simulink library "lib_Convection_FCConcCyls"  (R2015a)
settings: Solver=ode45  StartTime=0.0  StopTime=10.0  RelTol=1e-3
libraries: simulink x5, lib_Convection_NonDimParms x1
settings Model: Creator=jlkratz  LastModifiedBy=jlkratz

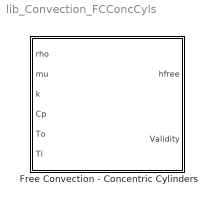
== system lib_Convection_FCConcCyls ==
  Free Convection - Concentric Cylinders : Subsystem  mask(TSAT: Concentric Cylinders Free Convection){R_M=1716, g_M=32.174, Ro_M=[1.5 5], Ri_M=[1 4], InOrOutSurf_M=Inner Surface}
      mask prompts: R_M "R_M - Real gas constant"; g_M "g_M - Acceleration due to gravity"; Ro_M "Ro_M - Radius of the outer cylinder"; Ri_M "Ri_M - Radius of the inner cylinder"; InOrOutSurf_M "InOrOutSurf_M - Select surface"
      mask help:
      | This block estimates the average convective heat transfer coefficient for free convection within concentric cylinders for either the inner or outer surface. The employed correlation is the work of Raithby and Hollands. Note that all fluid properrties should be evaluated at average of the hot and cold surface. To get the heat flux for the selected inner or outer surface, multiply the output (h) by the difference in temperature between the opposite surface and the selected surface. This number may be negative. Restrictions to the implemented correlation includes:
      |
      | 0.7 <= Pr <= 6000
      | Ra <= 10^7
      |
      | See the block help menu for more information.
      mask init:
      | %Initialization variables
      | 
      | %Characteristic length for Ra Calc
      | Lc_I = 2*log(Ro_M./Ri_M).^(4/3)./(Ri_M.^(-3/5) + Ro_M.^(-3/5)).^(5/3);
      mask Help: web(which('Convection_TSAT_FCConcCyls.html'),'-helpbrowser')
      mask TypeOptions InOrOutSurf_M: Inner Surface | Outer Surface

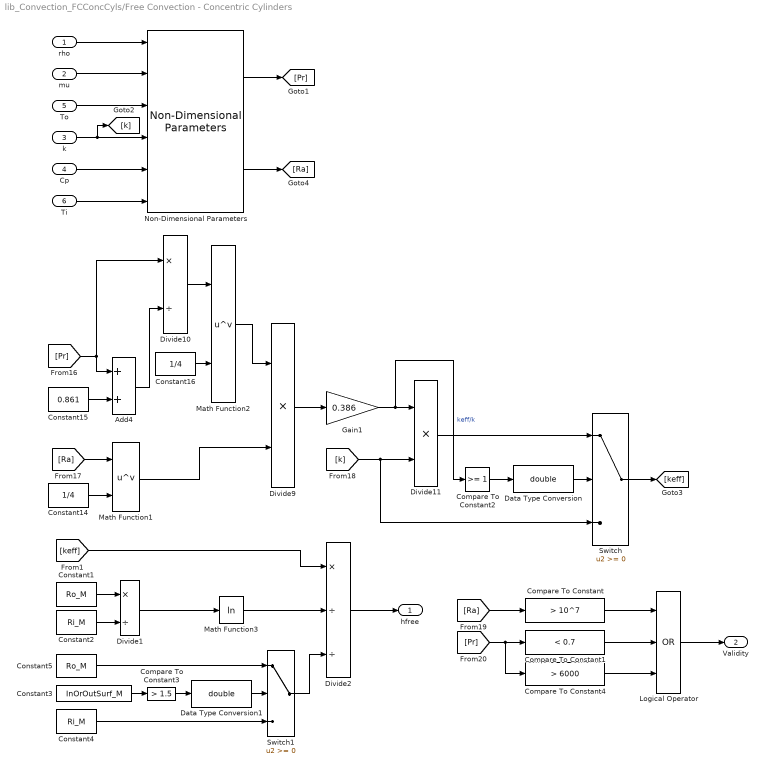
== system lib_Convection_FCConcCyls/Free Convection - Concentric Cylinders ==
  rho : Inport
  mu : Inport  Port=2
  k : Inport  Port=3
  Cp : Inport  Port=4
  To : Inport  Port=5
  Ti : Inport  Port=6
  Add4 : Sum
  Compare To Constant : simulink/Logic and Bit Operations/Compare To Constant  relop=>  const=10^7  OutDataTypeStr=boolean
  Compare To Constant1 : simulink/Logic and Bit Operations/Compare To Constant  relop=<  const=0.7  OutDataTypeStr=boolean
  Compare To Constant2 : simulink/Logic and Bit Operations/Compare To Constant  relop=>=  const=1  OutDataTypeStr=boolean
  Compare To Constant3 : simulink/Logic and Bit Operations/Compare To Constant  relop=>  const=1.5  OutDataTypeStr=boolean
  Compare To Constant4 : simulink/Logic and Bit Operations/Compare To Constant  relop=>  const=6000  OutDataTypeStr=boolean
  Constant1 : Constant  Value=Ro_M
  Constant14 : Constant  Value=1/4
  Constant15 : Constant  Value=0.861
  Constant16 : Constant  Value=1/4
  Constant2 : Constant  Value=Ri_M
  Constant3 : Constant  Value=InOrOutSurf_M
  Constant4 : Constant  Value=Ri_M
  Constant5 : Constant  Value=Ro_M
  Data Type Conversion : DataTypeConversion  OutDataTypeStr=double
  Data Type Conversion1 : DataTypeConversion  OutDataTypeStr=double
  Divide1 : Product  Inputs=*/
  Divide10 : Product  Inputs=*/
  Divide11 : Product  Inputs=**
  Divide2 : Product  Inputs=*//
  Divide9 : Product  Inputs=**
  Gain1 : Gain  Gain=0.386
  Logical Operator : Logic  Operator=OR  Inputs=3  AllPortsSameDT=off  OutDataTypeStr=boolean
  Math Function1 : Math  Operator=pow  SaturateOnIntegerOverflow=on
  Math Function2 : Math  Operator=pow  SaturateOnIntegerOverflow=on
  Math Function3 : Math  Operator=log  SaturateOnIntegerOverflow=on
  Non-Dimensional Parameters : lib_Convection_NonDimParms/Non-Dimensional Parameters  M_M=off  Re_M=off  Pr_M=on  Gr_M=off  Ra_M=on  Bi_M=off  Fo_M=off  Nu_M=off  St_M=off  Ec_M=off  jH_M=off  Pe_M=off  perfGas_M=on  R_M=R_M  mdot_A_or_rhov_M=off  A_M=1  L_M=Lc_I  g_M=g_M  t_M=1
  Switch : Switch
  Switch1 : Switch
  hfree : Outport
  Validity : Outport  Port=2
  wires:
  Compare To Constant4/1 -> Logical Operator/3
  Data Type Conversion1/1 -> Switch1/2
  Data Type Conversion/1 -> Switch/2
  rho/1 -> Non-Dimensional Parameters/1
  Compare To Constant3/1 -> Data Type Conversion1/1
  Compare To Constant1/1 -> Logical Operator/2
  Compare To Constant/1 -> Logical Operator/1
  Logical Operator/1 -> Validity/1
  [Ra] -> Compare To Constant/1
  [Pr] -> Compare To Constant1/1, Compare To Constant4/1
  Divide2/1 -> hfree/1
  [keff] -> Divide2/1
  Switch1/1 -> Divide2/3
  Math Function3/1 -> Divide2/2
  Constant5/1 -> Switch1/1
  Constant4/1 -> Switch1/3
  Constant3/1 -> Compare To Constant3/1
  Divide1/1 -> Math Function3/1
  Constant2/1 -> Divide1/2
  Constant1/1 -> Divide1/1
  Constant15/1 -> Add4/2
  Gain1/1 -> Divide11/1, Compare To Constant2/1  "keff/k"
  Math Function1/1 -> Divide9/2
  Add4/1 -> Divide10/2
  Math Function2/1 -> Divide9/1
  Divide9/1 -> Gain1/1
  [k] -> Switch/3, Divide11/2
  [Pr] -> Add4/1, Divide10/1
  Divide11/1 -> Switch/1
  Switch/1 -> [keff]
  Compare To Constant2/1 -> Data Type Conversion/1
  Divide10/1 -> Math Function2/1
  Constant16/1 -> Math Function2/2
  Constant14/1 -> Math Function1/2
  [Ra] -> Math Function1/1
  Non-Dimensional Parameters/1 -> [Pr]
  Non-Dimensional Parameters/2 -> [Ra]
  Cp/1 -> Non-Dimensional Parameters/5
  To/1 -> Non-Dimensional Parameters/3
  k/1 -> Non-Dimensional Parameters/4, [k]
  mu/1 -> Non-Dimensional Parameters/2
  Ti/1 -> Non-Dimensional Parameters/6
